simulink library "tqd"  (R2021b)
settings: Solver=VariableStepAuto  StartTime=0.0  StopTime=10.0  RelTol=1e-3
undefined symbols (not defined in the file or in its folder): ATQD_AccelLimitInRange_X_rpm, ATQD_AccelLimitInRange_Y_Nm, ATQD_AccelLimitOvrKi_X_Nm, ATQD_AccelLimitOvrKp_X_Nm, ATQD_BOSMapD_X_rpm, ATQD_BOSMapD_Y_pct, ATQD_BOSMapR_X_rpm, ATQD_BOSMapR_Y_pct, ATQD_HVBCurrSmooth_X_A, ATQD_LHMTqMapDLC_X_rpm, ATQD_LHMTqMapDLC_Y_pct, ATQD_LHMTqMapRLC_X_rpm, ATQD_LHMTqMapRLC_Y_pct, ATQD_NormalMapDLC_X_rpm, ATQD_NormalMapDLC_Y_pct, ATQD_NormalTqDecSR_X_rpm, ATQD_NormalTqDecSR_Y_Nm, ATQD_NormalTqIncSR_X_rpm, ATQD_NormalTqIncSR_Y_Nm, ATQD_OPDMapRLC_X_rpm, ATQD_OPDMapRLC_Y_pct, ATQD_RollRegTorReq_X_rpm, ATQD_RollRegTorReq_Y_enum, ATQD_VehSpdLimitInRange_X_rpm, ATQD_VehSpdLimitInRange_Y_Nm, ATQD_VehSpdLimitOvrKi_X_Nm, ATQD_VehSpdLimitOvrKp_X_Nm, EIGHT_INT, ENUM_BRAKEPEDAL_PRESSED, ENUM_BRAKEPEDAL_RELEASED, ENUM_COMBOKEY_DOWN, ENUM_COMBOKEY_M1, ENUM_COMBOKEY_M2, ENUM_COMBOKEY_NONE, ENUM_COMBOKEY_RKNEE, ENUM_COMBOKEY_STOPLV, ENUM_COMBOKEY_UP, ENUM_CP2VKNEEREQ_REQUEST, ENUM_CP2VNLVREQ_LEVEL1, ENUM_CP2VNLVREQ_LEVEL2, ENUM_CP2VNLVREQ_LOWER, ENUM_CP2VNLVREQ_STOPLV, ENUM_CP2VNLVREQ_UPPER, ENUM_CREEPIND_DISABLE, ENUM_CREEPIND_READY, ENUM_CREEPIND_RUNNING, ENUM_CREEPIND_WARNING, ENUM_DRIVELINERELEASE_RELEASE, ENUM_EBSTORQUERWQ_LIMIT, ENUM_EBSTORQUERWQ_TORQUE, ENUM_ECPVCUDRM_CONFORT, ENUM_ECPVCUDRM_ECO, ENUM_ECPVCUDRM_NORMAL, ENUM_ECPVCUDRM_NOTAVAILABLE, ENUM_EMTqModeDrvBrk_Accel, ENUM_EMTqModeDrvBrk_Brake, ENUM_EMTqModeDrvBrk_Coast, ENUM_ETC2ACTDRIVEDIR_BACKWARD, ENUM_ETC2ACTDRIVEDIR_FORWARD, ENUM_ETC2ACTDRIVEDIR_STILL ... (+341)
libraries: simulink x109, hcu_lib x67
(part 5 of 13)

== system tqd/TQD/OutpConvert/EVCU2 SCP ==
  BInpConvert_outputs : Inport
  Bus Selector1 : BusSelector  OutputSignals=VTQD_TMTqCapMot_Nm,VTQD_TMTqCapGen_Nm
  Constant1 : Constant  Value=EPS  OutDataTypeStr=single
  Constant143 : Constant  Value=KTQD_MCUMaxRefTorq_Nm
  Constant144 : Constant  Value=KTQD_MCUMaxRefTorq_Nm
  Constant5 : Constant  Value=EPS  OutDataTypeStr=single
  Data Type Conversion3 : DataTypeConversion  OutDataTypeStr=single
  Data Type Conversion96 : DataTypeConversion  OutDataTypeStr=single
  Divide4 : Product  Inputs=*/
  Divide5 : Product  Inputs=*/
  Fix4 : Rounding  Operator=round
  Fix5 : Rounding  Operator=round
  Gain1 : Gain  Gain=HUNDRED  ParamDataTypeStr=single
  Gain6 : Gain  Gain=HUNDRED  ParamDataTypeStr=single
  Max : MinMax  Function=max  Inputs=2
  Max1 : MinMax  Function=max  Inputs=2
  Saturation15 : Saturate  UpperLimit=100000  LowerLimit=1
      settings: AttributesFormatString=|
      | UpperLimit: %<UpperLimit>
      | LowerLimit: %<LowerLimit>
  Saturation16 : Saturate  UpperLimit=100000  LowerLimit=1
      settings: AttributesFormatString=|
      | UpperLimit: %<UpperLimit>
      | LowerLimit: %<LowerLimit>
  VTQD_EVCU2MaxTorqAvail_pct : Outport
  VTQD_EVCU2MinTorqAvail_pct : Outport  Port=2
  wires:
  Data Type Conversion96/1 -> [VTQD_EVCU2MaxTorqAvail_pct]  "VTQD_EVCU2MaxTorqAvail_pct"
  Data Type Conversion3/1 -> [VTQD_EVCU2MinTorqAvail_pct]  "VTQD_EVCU2MinTorqAvail_pct"
  Divide4/1 -> Gain6/1
  Fix5/1 -> Data Type Conversion3/1
  Constant144/1 -> Saturation16/1
  Fix4/1 -> Data Type Conversion96/1
  Gain6/1 -> Fix4/1
  Constant143/1 -> Saturation15/1
  BInpConvert_outputs/1 -> Bus Selector1/1
  Bus Selector1/1 -> [VTQD_TMTqCapMot_Nm]  "<VTQD_TMTqCapMot_Nm>"
  Bus Selector1/2 -> [VTQD_TMTqCapGen_Nm]  "<VTQD_TMTqCapGen_Nm>"
  Max/1 -> Divide4/2
  Saturation15/1 -> Max/1
  [VTQD_TMTqCapMot_Nm] -> Divide4/1
  Constant5/1 -> Max/2
  Saturation16/1 -> Max1/1
  Constant1/1 -> Max1/2
  Max1/1 -> Divide5/2
  [VTQD_TMTqCapGen_Nm] -> Divide5/1
  [VTQD_EVCU2MaxTorqAvail_pct] -> VTQD_EVCU2MaxTorqAvail_pct/1
  [VTQD_EVCU2MinTorqAvail_pct] -> VTQD_EVCU2MinTorqAvail_pct/1
  Divide5/1 -> Gain1/1
  Gain1/1 -> Fix5/1

== system tqd/TQD/OutpConvert/MCUCMD SCP ==
  BSCPIn_outputs : Inport
  BInpConvert_outputs : Inport  Port=2
  Bus Selector : BusSelector  OutputSignals=VTQD_BrkSWOn_flg
  Bus Selector1 : BusSelector  OutputSignals=VINP_TransReqGear_enum,VDMM_DTCDMSRCIncorrect_flg,VINP_CANMsgValidTC1_flg,VINP_ParkBrakeSW_flg
  Constant111 : Constant  Value=KTQD_VCUMCUDemSpd_rpm
  Constant14 : Constant  Value=ENUM_TARGETGEAR_REVERSE
  Constant156 : Constant  Value=ENUM_VCUMCUGEAR_D
  Constant157 : Constant  Value=ENUM_VCUMCUGEAR_R
  Constant159 : Constant  Value=ENUM_VCUMCUGEAR_N
  Constant190 : Constant  Value=ENUM_TARGETGEAR_NONE
  Constant191 : Constant  Value=ENUM_TARGETGEAR_NEUTRAL
  Constant192 : Constant  Value=ENUM_VCUMCUGEAR_INVAILD
  Constant5 : Constant  Value=ENUM_TARGETGEAR_DRIVE
  Constant58 : Constant  Value=KTQD_VCUMCUDemLoNegVal_rpm
  Constant66 : Constant  Value=ENUM_VCUMCUGEAR_N
  Constant89 : Constant  Value=ENUM_TARGETGEAR_ERROR
  Data Type Conversion : DataTypeConversion  OutDataTypeStr=boolean
  Data Type Conversion1 : DataTypeConversion  OutDataTypeStr=single
  Data Type Conversion2 : DataTypeConversion
  Data Type Conversion57 : DataTypeConversion  OutDataTypeStr=single
  Equal{22,24,27..29} (5 alike) : RelationalOperator  Operator===  OutDataTypeStr=boolean  RndMeth=Simplest
  NOT5 : Logic  Operator=NOT  AllPortsSameDT=off  OutDataTypeStr=boolean
  OR4 : Logic  Operator=OR  AllPortsSameDT=off  OutDataTypeStr=boolean
  OR5 : Logic  Operator=OR  AllPortsSameDT=off  OutDataTypeStr=boolean
  Switch{24,52..53,70..71} (5 alike) : Switch  Criteria=u2 ~= 0
      settings: AttributesFormatString=%<Criteria>
  Unit Delay2 : UnitDelay  InitialCondition=uint8(0)  SampleTime=-1  HasFrameUpgradeWarning=on
      settings: AttributesFormatString=%<InitialCondition>
  VTQD_VCUMCUDemLoNegVal_rpm : Outport
  VTQD_VCUMCUDemSpd_rpm : Outport  Port=2
  VTQD_VCUMCUGearSta_enum : Outport  Port=3
  VTQD_VCUMCUHandBrk_flg : Outport  Port=4
  VTQD_VCUMCUFootBrk_flg : Outport  Port=5
  wires:
  Switch52/1 -> Switch71/3
  Constant14/1 -> Equal24/2
  Equal29/1 -> OR4/2
  Equal22/1 -> Switch52/2
  Switch24/1 -> [VTQD_VCUMCUGearSta_enum], Unit Delay2/1  "VTQD_VCUMCUGearSta_enum"
  [VINP_TransReqGear_enum] -> Equal27/1
  Constant190/1 -> Equal28/2
  Equal27/1 -> OR5/2
  NOT5/1 -> OR5/1
  OR5/1 -> Switch71/2
  Equal28/1 -> OR4/1
  Constant5/1 -> Equal22/2
  Data Type Conversion57/1 -> [VTQD_VCUMCUDemSpd_rpm]  "VTQD_VCUMCUDemSpd_rpm"
  Constant191/1 -> Equal29/2
  [VINP_TransReqGear_enum] -> Equal29/1
  [VINP_CANMsgValidTC1_flg] -> NOT5/1
  [VINP_TransReqGear_enum] -> Equal22/1
  [VDMM_DTCDMSRCIncorrect_flg] -> Switch24/2
  Switch53/1 -> Switch52/3
  Constant111/1 -> Data Type Conversion57/1
  Switch71/1 -> Switch24/3
  Unit Delay2/1 -> Switch70/3
  Constant89/1 -> Equal27/2
  Constant156/1 -> Switch52/1
  Switch70/1 -> Switch53/3
  Constant159/1 -> Switch70/1
  OR4/1 -> Switch70/2
  Constant192/1 -> Switch71/1
  Equal24/1 -> Switch53/2
  [VINP_TransReqGear_enum] -> Equal28/1
  Constant58/1 -> Data Type Conversion1/1
  [VINP_TransReqGear_enum] -> Equal24/1
  Data Type Conversion1/1 -> [VTQD_VCUMCUDemLoNegVal_rpm]  "VTQD_VCUMCUDemLoNegVal_rpm"
  Constant157/1 -> Switch53/1
  Constant66/1 -> Switch24/1
  Bus Selector1/1 -> [VINP_TransReqGear_enum]  "<VINP_TransReqGear_enum>"
  BSCPIn_outputs/1 -> Bus Selector1/1
  Bus Selector1/2 -> [VDMM_DTCDMSRCIncorrect_flg]  "<VDMM_DTCDMSRCIncorrect_flg>"
  [VTQD_VCUMCUDemLoNegVal_rpm] -> VTQD_VCUMCUDemLoNegVal_rpm/1
  [VTQD_VCUMCUDemSpd_rpm] -> VTQD_VCUMCUDemSpd_rpm/1
  [VTQD_VCUMCUGearSta_enum] -> VTQD_VCUMCUGearSta_enum/1
  Bus Selector1/3 -> [VINP_CANMsgValidTC1_flg]  "<VINP_CANMsgValidTC1_flg>"
  Bus Selector1/4 -> [VINP_ParkBrakeSW_flg]  "<VINP_ParkBrakeSW_flg>"
  BInpConvert_outputs/1 -> Bus Selector/1
  Bus Selector/1 -> [VTQD_BrkSWOn_flg]  "<VTQD_BrkSWOn_flg>"
  [VINP_ParkBrakeSW_flg] -> Data Type Conversion/1
  Data Type Conversion/1 -> [VTQD_VCUMCUHandBrk_flg]  "VTQD_VCUMCUHandBrk_flg"
  [VTQD_BrkSWOn_flg] -> Data Type Conversion2/1
  Data Type Conversion2/1 -> [VTQD_VCUMCUFootBrk_flg]  "VTQD_VCUMCUFootBrk_flg"
  [VTQD_VCUMCUFootBrk_flg] -> VTQD_VCUMCUFootBrk_flg/1
  [VTQD_VCUMCUHandBrk_flg] -> VTQD_VCUMCUHandBrk_flg/1

== system tqd/TQD/OutpConvert/MSF SCP ==
  BInpConvert_outputs : Inport
  Bus Selector : BusSelector  OutputSignals=VTQD_ParkingProtectAction_flg
  Constant145 : Constant  Value=ENUM_VCUEBSHBSW_ACTIVE
  Constant181 : Constant  Value=ENUM_VCUEBSHBSW_PASSIVE
  Switch84 : Switch  Criteria=u2 ~= 0
      settings: AttributesFormatString=%<Criteria>
  VTQD_VCUEBSHBSw_enum : Outport
  wires:
  [VTQD_ParkingProtectAction_flg] -> Switch84/2
  Constant145/1 -> Switch84/1
  Switch84/1 -> [VTQD_VCUEBSHBSw_enum]  "VTQD_VCUEBSHBSw_enum"
  Constant181/1 -> Switch84/3
  BInpConvert_outputs/1 -> Bus Selector/1
  Bus Selector/1 -> [VTQD_ParkingProtectAction_flg]  "<VTQD_ParkingProtectAction_flg>"
  [VTQD_VCUEBSHBSw_enum] -> VTQD_VCUEBSHBSw_enum/1

== system tqd/TQD/OutpConvert/RC1 SCP ==
  Constant63 : Constant  Value=ZERO_INT  OutDataTypeStr=Inherit: Inherit via back propagation
  Constant64 : Constant  Value=FOUR_INT  OutDataTypeStr=single
  Constant65 : Constant  Value=KTQD_MCUMaxRefTorq_Nm
  Constant98 : Constant  Value=ZERO_FLOAT  OutDataTypeStr=single
  Data Type Conversion31 : DataTypeConversion  OutDataTypeStr=uint8
  Data Type Conversion32 : DataTypeConversion  OutDataTypeStr=uint8
  Data Type Conversion{33..43,58} (12 alike) : DataTypeConversion  OutDataTypeStr=single
  VTQD_RC1RetType_enum : Outport
  VTQD_RC1RetLocat_enum : Outport  Port=2
  VTQD_RC1RetCtrlMth_enum : Outport  Port=3
  VTQD_RC1RetSpdIdleP1_rpm : Outport  Port=4
  VTQD_RC1PctTrqIdleP1_pct : Outport  Port=5
  VTQD_RC1MaxRetSpdP2_rpm : Outport  Port=6
  VTQD_RC1RetSpdP2_pct : Outport  Port=7
  VTQD_RC1MaxRetSpdP3_rpm : Outport  Port=8
  VTQD_RC1PctTrqP3_pct : Outport  Port=9
  VTQD_RC1RetSpdP4_rpm : Outport  Port=10
  VTQD_RC1PctTrqP4_pct : Outport  Port=11
  VTQD_RC1RetSpdPekTrqP5_Nm : Outport  Port=12
  VTQD_RC1RefRetTrq_Nm : Outport  Port=13
  VTQD_RC1PctTrqPekTrqP5_pct : Outport  Port=14
  wires:
  Data Type Conversion33/1 -> VTQD_RC1RetCtrlMth_enum/1  "VTQD_RC1RetCtrlMth_enum"
  Data Type Conversion35/1 -> VTQD_RC1PctTrqIdleP1_pct/1  "VTQD_RC1PctTrqIdleP1_pct"
  Data Type Conversion32/1 -> VTQD_RC1RetLocat_enum/1  "VTQD_RC1RetLocat_enum"
  [DefaultValue16b] -> Data Type Conversion41/1
  [DefaultValue16b] -> Data Type Conversion34/1
  [DefaultValue16b] -> Data Type Conversion36/1
  Data Type Conversion39/1 -> VTQD_RC1RetSpdP4_rpm/1  "VTQD_RC1RetSpdP4_rpm"
  Data Type Conversion58/1 -> VTQD_RC1MaxRetSpdP3_rpm/1  "VTQD_RC1MaxRetSpdP3_rpm"
  [OfsetDefaultValue] -> Data Type Conversion37/1
  [OfsetDefaultValue] -> Data Type Conversion43/1
  Data Type Conversion42/1 -> VTQD_RC1RefRetTrq_Nm/1  "VTQD_RC1RefRetTrq_Nm"
  [OfsetDefaultValue] -> Data Type Conversion40/1
  [OfsetDefaultValue] -> Data Type Conversion38/1
  Data Type Conversion31/1 -> VTQD_RC1RetType_enum/1  "VTQD_RC1RetType_enum"
  Constant64/1 -> Data Type Conversion32/1
  Constant63/1 -> Data Type Conversion31/1
  [DefaultValue16b] -> Data Type Conversion39/1
  [DefaultValue8b] -> Data Type Conversion33/1
  [OfsetDefaultValue] -> Data Type Conversion35/1
  Data Type Conversion36/1 -> VTQD_RC1MaxRetSpdP2_rpm/1  "VTQD_RC1MaxRetSpdP2_rpm"
  [DefaultValue16b] -> Data Type Conversion58/1
  Data Type Conversion40/1 -> VTQD_RC1PctTrqP4_pct/1  "VTQD_RC1PctTrqP4_pct"
  Data Type Conversion38/1 -> VTQD_RC1PctTrqP3_pct/1  "VTQD_RC1PctTrqP3_pct"
  Data Type Conversion41/1 -> VTQD_RC1RetSpdPekTrqP5_Nm/1  "VTQD_RC1RetSpdPekTrqP5_Nm"
  Data Type Conversion37/1 -> VTQD_RC1RetSpdP2_pct/1  "VTQD_RC1RetSpdP2_pct"
  Data Type Conversion43/1 -> VTQD_RC1PctTrqPekTrqP5_pct/1  "VTQD_RC1PctTrqPekTrqP5_pct"
  Constant65/1 -> Data Type Conversion42/1
  Data Type Conversion34/1 -> VTQD_RC1RetSpdIdleP1_rpm/1  "VTQD_RC1RetSpdIdleP1_rpm"
  Constant98/1 -> [OfsetDefaultValue], [DefaultValue8b], [DefaultValue16b]

== system tqd/TQD/OutpConvert/TUpA Indication ==
  BInpConvert_outputs : Inport
  Bus Selector : BusSelector  OutputSignals=VTQD_ComboKeyEn_flg,VTQD_ActTUpAIND_enum
  Constant19 : Constant  Value=ENUM_TUPAIND_RUNNING
  Switch1 : Switch  Criteria=u2 ~= 0
      settings: AttributesFormatString=%<Criteria>
  VTQD_TUpAIND_enum : Outport
  wires:
  Constant19/1 -> Switch1/1
  [VTQD_ActTUpAIND_enum] -> Switch1/3
  Switch1/1 -> [VTQD_TUpAIND_enum]  "VTQD_TUpAIND_enum"
  [VTQD_ComboKeyEn_flg] -> Switch1/2
  Bus Selector/1 -> [VTQD_ComboKeyEn_flg]  "<VTQD_ComboKeyEn_flg>"
  BInpConvert_outputs/1 -> Bus Selector/1
  Bus Selector/2 -> [VTQD_ActTUpAIND_enum]  "<VTQD_ActTUpAIND_enum>"
  [VTQD_TUpAIND_enum] -> VTQD_TUpAIND_enum/1

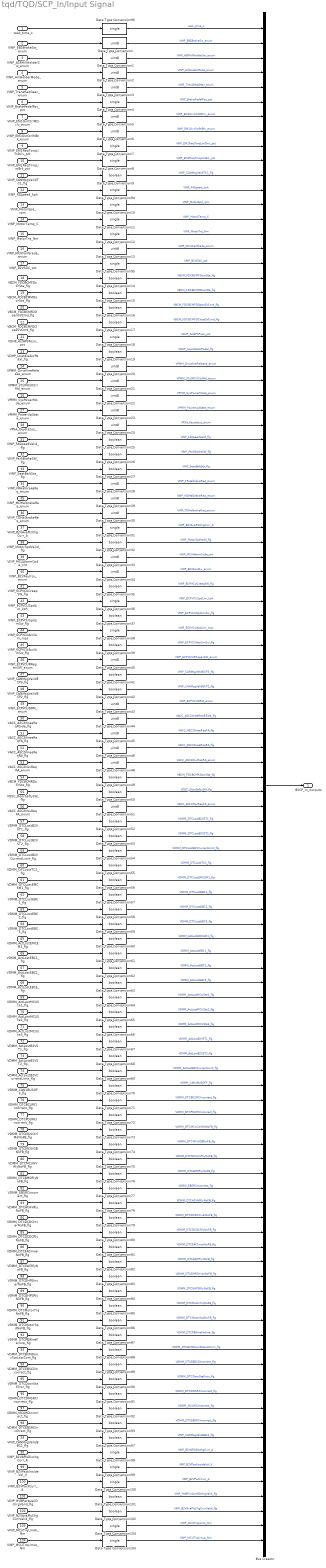
== system tqd/TQD/SCP_In/Input Signal ==
  task_time_s : Inport
  VINP_EBSBrakeSw_enum : Inport  Port=2
  VINP_ASRHillHolderSw_enum : Inport  Port=3
  VINP_HillHolderMode_enum : Inport  Port=4
  VINP_TransReqGear_enum : Inport  Port=5
  VINP_BrakePedalPos_pct : Inport  Port=6
  VINP_EM1OvrCtrlMDriv_enum : Inport  Port=7
  VINP_EM1OvrCtrlMBrk_enum : Inport  Port=8
  VINP_EM1ReqTorqLimDriv_pct : Inport  Port=9
  VINP_EM1ReqTorqLimBrk_pct : Inport  Port=10
  VINP_CANMsgValidTC1_flg : Inport  Port=11
  VINP_FASpeed_kph : Inport  Port=12
  VINP_MotorSpd_rpm : Inport  Port=13
  VINP_MotorTemp_C : Inport  Port=14
  VINP_MotorTrq_Nm : Inport  Port=15
  VINP_MCUFailGrade_enum : Inport  Port=16
  VINP_B2VSOC_pct : Inport  Port=17
  VBCM_FDCBCMFDoorSta_flg : Inport  Port=18
  VBCM_FDCBCMMDoorSta_flg : Inport  Port=19
  VBCM_FDCBCMFDOpenSVCmd_flg : Inport  Port=20
  VBCM_FDCBCMFDCloseSVCmd_flg : Inport  Port=21
  VDHP_ActAPSPosn_pct : Inport  Port=22
  VDHP_LowIdleAccPedal_flg : Inport  Port=23
  VPMM_DrivelineRelease_enum : Inport  Port=24
  VPMM_VCUMCUCtrlMd_enum : Inport  Port=25
  VPMM_SysPowerMode_enum : Inport  Port=26
  VPMM_PowerUpState_enum : Inport  Port=27
  VPSA_Keystatus_enum : Inport  Port=28
  VINP_CANMsgValidEBC2_flg : Inport  Port=29
  VINP_B2VAPlsDischgCurr_A : Inport  Port=30
  VINP_FASpeedValid_flg : Inport  Port=31
  VINP_ParkBrakeSW_flg : Inport  Port=32
  VINP_SeatBeltSta_flg : Inport  Port=33
  VINP_FRHalbrakeReq_enum : Inport  Port=34
  VINP_MDHalbrakeReq_enum : Inport  Port=35
  VINP_TDHalbrakeReq_enum : Inport  Port=36
  VINP_B2VAvaPlsChgCurr_A : Inport  Port=37
  VINP_MotorSpdValid_flg : Inport  Port=38
  VINP_MCUAlarmCode_cnt : Inport  Port=39
  VINP_B2VFaultLv_enum : Inport  Port=40
  VINP_ECPVCUCreepSW_flg : Inport  Port=41
  VINP_ECPVCUSpdLim_kph : Inport  Port=42
  VINP_ECPVCUSpdLimSw_flg : Inport  Port=43
  VINP_ECPVCUAcclLim_mps : Inport  Port=44
  VINP_ECPVCUAcclLimSw_flg : Inport  Port=45
  VINP_ECPVCURRegenSW_enum : Inport  Port=46
  VINP_CANMsgValidECP3_flg : Inport  Port=47
  VINP_CANMsgValidECP2_flg : Inport  Port=48
  VINP_ECPVCUDRM_enum : Inport  Port=49
  VACC_ASC2KneeReqRSide_flg : Inport  Port=50
  VACC_ASC2KneeReqFA_flg : Inport  Port=51
  VACC_ASC2KneeReqRA_flg : Inport  Port=52
  VACC_ASC2NLvReqRA_enum : Inport  Port=53
  VBCM_FDCBCMRDoorSta_flg : Inport  Port=54
  VDSC_DoorSaftySW_flg : Inport  Port=55
  VACC_ASC2NLvReqFA_enum : Inport  Port=56
  VDMM_DTCLostB2VST1_flg : Inport  Port=57
  VDMM_DTCLostB2VST2_flg : Inport  Port=58
  VDMM_DTCLostB2VCurrentLimit_flg : Inport  Port=59
  VDMM_DTCLostTC1_flg : Inport  Port=60
  VDMM_DTCLostEMCEM1_flg : Inport  Port=61
  VDMM_DTCLostEBC1_flg : Inport  Port=62
  VDMM_DTCLostEBC2_flg : Inport  Port=63
  VDMM_DTCLostEBC5_flg : Inport  Port=64
  VDMM_ActLostEMCEM1_flg : Inport  Port=65
  VDMM_ActLostEBC1_flg : Inport  Port=66
  VDMM_ActLostEBC2_flg : Inport  Port=67
  VDMM_ActLostEBC5_flg : Inport  Port=68
  VDMM_ActLostMCUSta1_flg : Inport  Port=69
  VDMM_ActLostMCUSta2_flg : Inport  Port=70
  VDMM_ActLostMCUSta3_flg : Inport  Port=71
  VDMM_ActLostB2VST1_flg : Inport  Port=72
  VDMM_ActLostB2VST2_flg : Inport  Port=73
  VDMM_ActLostB2VCurrentLimit_flg : Inport  Port=74
  VDMM_CAN1BUSOFF_flg : Inport  Port=75
  VDMM_DTCBCURCIncorrect_flg : Inport  Port=76
  VDMM_DTCPDURCIncorrect_flg : Inport  Port=77
  VDMM_DTCMCUCtrlMdNoFB_flg : Inport  Port=78
  VDMM_DTCMCUIGBNoFB_flg : Inport  Port=79
  VDMM_DTCMCUHVRlyNoFB_flg : Inport  Port=80
  VDMM_DTCBMSRlyNoFB_flg : Inport  Port=81
  VDMM_EBSRCIncorrect_flg : Inport  Port=82
  VDMM_DTCACHVRlyNoFB_flg : Inport  Port=83
  VDMM_DTCDCDCInverNoFB_flg : Inport  Port=84
  VDMM_DTCDCDCRlyNoFB_flg : Inport  Port=85
  VDMM_DTCEACInverNoFB_flg : Inport  Port=86
  VDMM_DTCEACRlyNoFB_flg : Inport  Port=87
  VDMM_DTCEHPSInverNoFB_flg : Inport  Port=88
  VDMM_DTCEHPSRlyNoFB_flg : Inport  Port=89
  VDMM_DTCMotorTrqNoFB_flg : Inport  Port=90
  VDMM_DTCMotorSpdNoFB_flg : Inport  Port=91
  VDMM_DTCPBWireFailure_flg : Inport  Port=92
  VDMM_DTCBCMDoorStaLostCom_flg : Inport  Port=93
  VDMM_DTCEBSCSIncorrect_flg : Inport  Port=94
  VDMM_DTCDoorStaError_flg : Inport  Port=95
  VDMM_DTCDMSRCIncorrect_flg : Inport  Port=96
  VDMM_MCURCIncorrect_flg : Inport  Port=97
  VDMM_DTCEBSRCIncorrect_flg : Inport  Port=98
  VINP_B2VPackInsideVol_V : Inport  Port=99
  VINP_B2VPackCurr_A : Inport  Port=100
  VINP_HVBPwrAvailDchrgValid_flg : Inport  Port=101
  VINP_B2VAvaPlsChgCurrValid_flg : Inport  Port=102
  VINP_MCUTrqLimHi_Nm : Inport  Port=103
  VINP_MCUTrqLimLo_Nm : Inport  Port=104
  Bus Creator : BusCreator  Inputs=104
  Data Type Conversion{,1..3,5..6,13,20..24,28..30,33..34,40,43..46,48,51} (24 alike) : DataTypeConversion  OutDataTypeStr=uint8
  Data Type Conversion{4,7..8,10..12,18,31,36,38,94..96,98..100,103..104} (18 alike) : DataTypeConversion  OutDataTypeStr=single
  Data Type Conversion{9,14..17,19,25..27,32,35,37,39,41..42,49..50,52..93,97,101..102} (62 alike) : DataTypeConversion  OutDataTypeStr=boolean
  BSCP_In_outputs : Outport
  wires:
  VINP_ECPVCUAcclLim_mps/1 -> Data Type Conversion38/1
  VDMM_DTCBCMDoorStaLostCom_flg/1 -> Data Type Conversion88/1
  Data Type Conversion30/1 -> Bus Creator/34  "VINP_TDHalbrakeReq_enum"
  VINP_SeatBeltSta_flg/1 -> Data Type Conversion27/1
  Data Type Conversion29/1 -> Bus Creator/33  "VINP_MDHalbrakeReq_enum"
  VINP_MDHalbrakeReq_enum/1 -> Data Type Conversion29/1
  Data Type Conversion94/1 -> Bus Creator/12  "VINP_FASpeed_kph"
  VDMM_DTCDCDCRlyNoFB_flg/1 -> Data Type Conversion80/1
  Data Type Conversion20/1 -> Bus Creator/24  "VPMM_DrivelineRelease_enum"
  VDMM_DTCDoorStaError_flg/1 -> Data Type Conversion90/1
  Data Type Conversion14/1 -> Bus Creator/18  "VBCM_FDCBCMFDoorSta_flg"
  Data Type Conversion3/1 -> Bus Creator/5  "VINP_TransReqGear_enum"
  VINP_EBSBrakeSw_enum/1 -> Data Type Conversion/1
  Data Type Conversion6/1 -> Bus Creator/8  "VINP_EM1OvrCtrlMBrk_enum"
  VINP_EM1OvrCtrlMBrk_enum/1 -> Data Type Conversion6/1
  VPMM_SysPowerMode_enum/1 -> Data Type Conversion22/1
  Data Type Conversion38/1 -> Bus Creator/42  "VINP_ECPVCUAcclLim_mps"
  VDMM_DTCDCDCInverNoFB_flg/1 -> Data Type Conversion79/1
  Data Type Conversion43/1 -> Bus Creator/47  "VINP_ECPVCUDRM_enum"
  Data Type Conversion18/1 -> Bus Creator/22  "VDHP_ActAPSPosn_pct"
  Data Type Conversion46/1 -> Bus Creator/50  "VACC_ASC2KneeReqRA_flg"
  Data Type Conversion16/1 -> Bus Creator/20  "VBCM_FDCBCMFDOpenSVCmd_flg"
  VPSA_Keystatus_enum/1 -> Data Type Conversion24/1
  VDMM_DTCMotorSpdNoFB_flg/1 -> Data Type Conversion86/1
  Data Type Conversion45/1 -> Bus Creator/49  "VACC_ASC2KneeReqFA_flg"
  VDMM_DTCPDURCIncorrect_flg/1 -> Data Type Conversion72/1
  Data Type Conversion5/1 -> Bus Creator/7  "VINP_EM1OvrCtrlMDriv_enum"
  Data Type Conversion22/1 -> Bus Creator/26  "VPMM_SysPowerMode_enum"
  VDMM_ActLostEBC1_flg/1 -> Data Type Conversion61/1
  Data Type Conversion35/1 -> Bus Creator/39  "VINP_ECPVCUCreepSW_flg"
  VINP_MCUAlarmCode_cnt/1 -> Data Type Conversion33/1
  Data Type Conversion34/1 -> Bus Creator/38  "VINP_B2VFaultLv_enum"
  Data Type Conversion19/1 -> Bus Creator/23  "VDHP_LowIdleAccPedal_flg"
  Data Type Conversion1/1 -> Bus Creator/3  "VINP_ASRHillHolderSw_enum"
  Data Type Conversion15/1 -> Bus Creator/19  "VBCM_FDCBCMMDoorSta_flg"
  VINP_CANMsgValidECP2_flg/1 -> Data Type Conversion42/1
  VDSC_DoorSaftySW_flg/1 -> Data Type Conversion50/1
  Data Type Conversion33/1 -> Bus Creator/37  "VINP_MCUAlarmCode_cnt"
  Data Type Conversion96/1 -> Bus Creator/1  "task_time_s"
  VDMM_DTCEHPSInverNoFB_flg/1 -> Data Type Conversion83/1
  VINP_FASpeed_kph/1 -> Data Type Conversion94/1
  VACC_ASC2NLvReqRA_enum/1 -> Data Type Conversion48/1
  VINP_ECPVCUSpdLim_kph/1 -> Data Type Conversion36/1
  Data Type Conversion12/1 -> Bus Creator/15  "VINP_MotorTrq_Nm"
  VINP_HillHolderMode_enum/1 -> Data Type Conversion2/1
  VDHP_LowIdleAccPedal_flg/1 -> Data Type Conversion19/1
  Data Type Conversion36/1 -> Bus Creator/40  "VINP_ECPVCUSpdLim_kph"
  Data Type Conversion37/1 -> Bus Creator/41  "VINP_ECPVCUSpdLimSw_flg"
  Data Type Conversion17/1 -> Bus Creator/21  "VBCM_FDCBCMFDCloseSVCmd_flg"
  Data Type Conversion4/1 -> Bus Creator/6  "VINP_BrakePedalPos_pct"
  VDMM_MCURCIncorrect_flg/1 -> Data Type Conversion92/1
  Data Type Conversion9/1 -> Bus Creator/11  "VINP_CANMsgValidTC1_flg"
  Data Type Conversion95/1 -> Bus Creator/17  "VINP_B2VSOC_pct"
  Data Type Conversion21/1 -> Bus Creator/25  "VPMM_VCUMCUCtrlMd_enum"
  Data Type Conversion42/1 -> Bus Creator/46  "VINP_CANMsgValidECP2_flg"
  Data Type Conversion39/1 -> Bus Creator/43  "VINP_ECPVCUAcclLimSw_flg"
  Data Type Conversion28/1 -> Bus Creator/32  "VINP_FRHalbrakeReq_enum"
  VBCM_FDCBCMFDCloseSVCmd_flg/1 -> Data Type Conversion17/1
  Data Type Conversion8/1 -> Bus Creator/10  "VINP_EM1ReqTorqLimBrk_pct"
  Data Type Conversion40/1 -> Bus Creator/44  "VINP_ECPVCURRegenSW_enum"
  VDMM_DTCEACRlyNoFB_flg/1 -> Data Type Conversion82/1
  Data Type Conversion/1 -> Bus Creator/2  "VINP_EBSBrakeSw_enum"
  VBCM_FDCBCMFDoorSta_flg/1 -> Data Type Conversion14/1
  Data Type Conversion24/1 -> Bus Creator/28  "VPSA_Keystatus_enum"
  Data Type Conversion23/1 -> Bus Creator/27  "VPMM_PowerUpState_enum"
  Data Type Conversion7/1 -> Bus Creator/9  "VINP_EM1ReqTorqLimDriv_pct"
  Data Type Conversion32/1 -> Bus Creator/36  "VINP_MotorSpdValid_flg"
  Data Type Conversion10/1 -> Bus Creator/13  "VINP_MotorSpd_rpm"
  VDMM_CAN1BUSOFF_flg/1 -> Data Type Conversion70/1
  Data Type Conversion44/1 -> Bus Creator/48  "VACC_ASC2KneeReqRSide_flg"
  VINP_ASRHillHolderSw_enum/1 -> Data Type Conversion1/1
  VINP_ECPVCUDRM_enum/1 -> Data Type Conversion43/1
  VBCM_FDCBCMMDoorSta_flg/1 -> Data Type Conversion15/1
  Data Type Conversion31/1 -> Bus Creator/35  "VINP_B2VAvaPlsChgCurr_A"
  Data Type Conversion26/1 -> Bus Creator/30  "VINP_ParkBrakeSW_flg"
  Data Type Conversion25/1 -> Bus Creator/29  "VINP_FASpeedValid_flg"
  Data Type Conversion41/1 -> Bus Creator/45  "VINP_CANMsgValidECP3_flg"
  VINP_ECPVCUSpdLimSw_flg/1 -> Data Type Conversion37/1
  Data Type Conversion27/1 -> Bus Creator/31  "VINP_SeatBeltSta_flg"
  Bus Creator/1 -> BSCP_In_outputs/1
  Data Type Conversion11/1 -> Bus Creator/14  "VINP_MotorTemp_C"
  Data Type Conversion2/1 -> Bus Creator/4  "VINP_HillHolderMode_enum"
  Data Type Conversion13/1 -> Bus Creator/16  "VINP_MCUFailGrade_enum"
  VDMM_DTCMCUCtrlMdNoFB_flg/1 -> Data Type Conversion73/1
  VINP_ParkBrakeSW_flg/1 -> Data Type Conversion26/1
  VDMM_DTCMCUHVRlyNoFB_flg/1 -> Data Type Conversion75/1
  VDMM_DTCLostB2VST2_flg/1 -> Data Type Conversion53/1
  VDMM_ActLostMCUSta3_flg/1 -> Data Type Conversion66/1
  VDMM_ActLostEMCEM1_flg/1 -> Data Type Conversion60/1
  VBCM_FDCBCMRDoorSta_flg/1 -> Data Type Conversion49/1
  VINP_TransReqGear_enum/1 -> Data Type Conversion3/1
  VACC_ASC2KneeReqRA_flg/1 -> Data Type Conversion46/1
  VDMM_DTCEBSCSIncorrect_flg/1 -> Data Type Conversion89/1
  VINP_EM1ReqTorqLimBrk_pct/1 -> Data Type Conversion8/1
  VINP_EM1ReqTorqLimDriv_pct/1 -> Data Type Conversion7/1
  VPMM_DrivelineRelease_enum/1 -> Data Type Conversion20/1
  VDMM_DTCDMSRCIncorrect_flg/1 -> Data Type Conversion91/1
  VINP_FRHalbrakeReq_enum/1 -> Data Type Conversion28/1
  VDMM_DTCMCUIGBNoFB_flg/1 -> Data Type Conversion74/1
  VINP_EM1OvrCtrlMDriv_enum/1 -> Data Type Conversion5/1
  VINP_MotorSpdValid_flg/1 -> Data Type Conversion32/1
  VINP_ECPVCUCreepSW_flg/1 -> Data Type Conversion35/1
  VDMM_DTCLostEBC1_flg/1 -> Data Type Conversion57/1
  VDMM_ActLostB2VST2_flg/1 -> Data Type Conversion68/1
  VINP_FASpeedValid_flg/1 -> Data Type Conversion25/1
  VDMM_DTCEHPSRlyNoFB_flg/1 -> Data Type Conversion84/1
  VDMM_DTCMotorTrqNoFB_flg/1 -> Data Type Conversion85/1
  VINP_CANMsgValidTC1_flg/1 -> Data Type Conversion9/1
  VDMM_DTCEBSRCIncorrect_flg/1 -> Data Type Conversion93/1
  VDMM_DTCPBWireFailure_flg/1 -> Data Type Conversion87/1
  VPMM_PowerUpState_enum/1 -> Data Type Conversion23/1
  VPMM_VCUMCUCtrlMd_enum/1 -> Data Type Conversion21/1
  VINP_B2VSOC_pct/1 -> Data Type Conversion95/1
  VDMM_EBSRCIncorrect_flg/1 -> Data Type Conversion77/1
  VDMM_ActLostB2VCurrentLimit_flg/1 -> Data Type Conversion69/1
  VACC_ASC2KneeReqRSide_flg/1 -> Data Type Conversion44/1
  VACC_ASC2KneeReqFA_flg/1 -> Data Type Conversion45/1
  VDMM_DTCLostB2VST1_flg/1 -> Data Type Conversion52/1
  VDMM_DTCACHVRlyNoFB_flg/1 -> Data Type Conversion78/1
  VDMM_DTCLostTC1_flg/1 -> Data Type Conversion55/1
  VINP_ECPVCUAcclLimSw_flg/1 -> Data Type Conversion39/1
  VINP_CANMsgValidECP3_flg/1 -> Data Type Conversion41/1
  VDMM_DTCLostEBC2_flg/1 -> Data Type Conversion58/1
  VACC_ASC2NLvReqFA_enum/1 -> Data Type Conversion51/1
  VINP_B2VAvaPlsChgCurr_A/1 -> Data Type Conversion31/1
  VDMM_ActLostMCUSta2_flg/1 -> Data Type Conversion65/1
  VDMM_ActLostEBC2_flg/1 -> Data Type Conversion62/1
  VDMM_ActLostMCUSta1_flg/1 -> Data Type Conversion64/1
  VDMM_ActLostB2VST1_flg/1 -> Data Type Conversion67/1
  VINP_MCUFailGrade_enum/1 -> Data Type Conversion13/1
  VDMM_DTCLostEBC5_flg/1 -> Data Type Conversion59/1
  VBCM_FDCBCMFDOpenSVCmd_flg/1 -> Data Type Conversion16/1
  VDHP_ActAPSPosn_pct/1 -> Data Type Conversion18/1
  VDMM_ActLostEBC5_flg/1 -> Data Type Conversion63/1
  VINP_BrakePedalPos_pct/1 -> Data Type Conversion4/1
  VDMM_DTCBCURCIncorrect_flg/1 -> Data Type Conversion71/1
  VINP_B2VFaultLv_enum/1 -> Data Type Conversion34/1
  VDMM_DTCEACInverNoFB_flg/1 -> Data Type Conversion81/1
  VINP_TDHalbrakeReq_enum/1 -> Data Type Conversion30/1
  VDMM_DTCLostEMCEM1_flg/1 -> Data Type Conversion56/1
  VINP_MotorSpd_rpm/1 -> Data Type Conversion10/1
  VINP_ECPVCURRegenSW_enum/1 -> Data Type Conversion40/1
  VINP_MotorTemp_C/1 -> Data Type Conversion11/1
  VDMM_DTCLostB2VCurrentLimit_flg/1 -> Data Type Conversion54/1
  VDMM_DTCBMSRlyNoFB_flg/1 -> Data Type Conversion76/1
  VINP_MotorTrq_Nm/1 -> Data Type Conversion12/1
  task_time_s/1 -> Data Type Conversion96/1
  VINP_CANMsgValidEBC2_flg/1 -> Data Type Conversion97/1
  VINP_B2VAPlsDischgCurr_A/1 -> Data Type Conversion98/1
  VINP_B2VAvaPlsChgCurrValid_flg/1 -> Data Type Conversion102/1
  VINP_HVBPwrAvailDchrgValid_flg/1 -> Data Type Conversion101/1
  VINP_B2VPackInsideVol_V/1 -> Data Type Conversion99/1
  VINP_B2VPackCurr_A/1 -> Data Type Conversion100/1
  VINP_MCUTrqLimLo_Nm/1 -> Data Type Conversion103/1
  VINP_MCUTrqLimHi_Nm/1 -> Data Type Conversion104/1
  Data Type Conversion48/1 -> Bus Creator/51  "VACC_ASC2NLvReqRA_enum"
  Data Type Conversion49/1 -> Bus Creator/52  "VBCM_FDCBCMRDoorSta_flg"
  Data Type Conversion50/1 -> Bus Creator/53  "VDSC_DoorSaftySW_flg"
  Data Type Conversion51/1 -> Bus Creator/54  "VACC_ASC2NLvReqFA_enum"
  Data Type Conversion52/1 -> Bus Creator/55  "VDMM_DTCLostB2VST1_flg"
  Data Type Conversion53/1 -> Bus Creator/56  "VDMM_DTCLostB2VST2_flg"
  Data Type Conversion54/1 -> Bus Creator/57  "VDMM_DTCLostB2VCurrentLimit_flg"
  Data Type Conversion55/1 -> Bus Creator/58  "VDMM_DTCLostTC1_flg"
  Data Type Conversion56/1 -> Bus Creator/59  "VDMM_DTCLostEMCEM1_flg"
  Data Type Conversion57/1 -> Bus Creator/60  "VDMM_DTCLostEBC1_flg"
  Data Type Conversion58/1 -> Bus Creator/61  "VDMM_DTCLostEBC2_flg"
  Data Type Conversion59/1 -> Bus Creator/62  "VDMM_DTCLostEBC5_flg"
  Data Type Conversion60/1 -> Bus Creator/63  "VDMM_ActLostEMCEM1_flg"
  Data Type Conversion61/1 -> Bus Creator/64  "VDMM_ActLostEBC1_flg"
  Data Type Conversion62/1 -> Bus Creator/65  "VDMM_ActLostEBC2_flg"
  Data Type Conversion63/1 -> Bus Creator/66  "VDMM_ActLostEBC5_flg"
  Data Type Conversion64/1 -> Bus Creator/67  "VDMM_ActLostMCUSta1_flg"
  Data Type Conversion65/1 -> Bus Creator/68  "VDMM_ActLostMCUSta2_flg"
  Data Type Conversion66/1 -> Bus Creator/69  "VDMM_ActLostMCUSta3_flg"
  Data Type Conversion67/1 -> Bus Creator/70  "VDMM_ActLostB2VST1_flg"
  Data Type Conversion68/1 -> Bus Creator/71  "VDMM_ActLostB2VST2_flg"
  Data Type Conversion69/1 -> Bus Creator/72  "VDMM_ActLostB2VCurrentLimit_flg"
  Data Type Conversion70/1 -> Bus Creator/73  "VDMM_CAN1BUSOFF_flg"
  Data Type Conversion71/1 -> Bus Creator/74  "VDMM_DTCBCURCIncorrect_flg"
  Data Type Conversion72/1 -> Bus Creator/75  "VDMM_DTCPDURCIncorrect_flg"
  Data Type Conversion73/1 -> Bus Creator/76  "VDMM_DTCMCUCtrlMdNoFB_flg"
  Data Type Conversion74/1 -> Bus Creator/77  "VDMM_DTCMCUIGBNoFB_flg"
  Data Type Conversion75/1 -> Bus Creator/78  "VDMM_DTCMCUHVRlyNoFB_flg"
  Data Type Conversion76/1 -> Bus Creator/79  "VDMM_DTCBMSRlyNoFB_flg"
  Data Type Conversion77/1 -> Bus Creator/80  "VDMM_EBSRCIncorrect_flg"
  Data Type Conversion78/1 -> Bus Creator/81  "VDMM_DTCACHVRlyNoFB_flg"
  Data Type Conversion79/1 -> Bus Creator/82  "VDMM_DTCDCDCInverNoFB_flg"
  Data Type Conversion80/1 -> Bus Creator/83  "VDMM_DTCDCDCRlyNoFB_flg"
  Data Type Conversion81/1 -> Bus Creator/84  "VDMM_DTCEACInverNoFB_flg"
  Data Type Conversion82/1 -> Bus Creator/85  "VDMM_DTCEACRlyNoFB_flg"
  Data Type Conversion83/1 -> Bus Creator/86  "VDMM_DTCEHPSInverNoFB_flg"
  Data Type Conversion84/1 -> Bus Creator/87  "VDMM_DTCEHPSRlyNoFB_flg"
  Data Type Conversion85/1 -> Bus Creator/88  "VDMM_DTCMotorTrqNoFB_flg"
  Data Type Conversion86/1 -> Bus Creator/89  "VDMM_DTCMotorSpdNoFB_flg"
  Data Type Conversion87/1 -> Bus Creator/90  "VDMM_DTCPBWireFailure_flg"
  Data Type Conversion88/1 -> Bus Creator/91  "VDMM_DTCBCMDoorStaLostCom_flg"
  Data Type Conversion89/1 -> Bus Creator/92  "VDMM_DTCEBSCSIncorrect_flg"
  Data Type Conversion90/1 -> Bus Creator/93  "VDMM_DTCDoorStaError_flg"
  Data Type Conversion91/1 -> Bus Creator/94  "VDMM_DTCDMSRCIncorrect_flg"
  Data Type Conversion92/1 -> Bus Creator/95  "VDMM_MCURCIncorrect_flg"
  Data Type Conversion93/1 -> Bus Creator/96  "VDMM_DTCEBSRCIncorrect_flg"
  Data Type Conversion97/1 -> Bus Creator/97  "VINP_CANMsgValidEBC2_flg"
  Data Type Conversion98/1 -> Bus Creator/98  "VINP_B2VAPlsDischgCurr_A"
  Data Type Conversion99/1 -> Bus Creator/99  "VINP_B2VPackInsideVol_V"
  Data Type Conversion100/1 -> Bus Creator/100  "VINP_B2VPackCurr_A"
  Data Type Conversion101/1 -> Bus Creator/101  "VINP_HVBPwrAvailDchrgValid_flg"
  Data Type Conversion102/1 -> Bus Creator/102  "VINP_B2VAvaPlsChgCurrValid_flg"
  Data Type Conversion104/1 -> Bus Creator/103  "VINP_MCUTrqLimHi_Nm"
  Data Type Conversion103/1 -> Bus Creator/104  "VINP_MCUTrqLimLo_Nm"

== system tqd/TQD/SCP_In/Invalid Condition ==
  VDMM_MCURCIncorrect_flg : Inport
  VINP_FASpeedValid_flg : Inport  Port=2
  VDMM_DTCDMSRCIncorrect_flg : Inport  Port=3
  VDMM_DTCEBSRCIncorrect_flg : Inport  Port=4
  VINP_MotorSpdValid_flg : Inport  Port=5
  Bus Creator : BusCreator  Inputs=10
  Data Type Conversion{,1..9} (10 alike) : DataTypeConversion  OutDataTypeStr=boolean
  NOT : Logic  Operator=NOT  AllPortsSameDT=off  OutDataTypeStr=boolean
  NOT1 : Logic  Operator=NOT  AllPortsSameDT=off  OutDataTypeStr=boolean
  OR : Logic  Operator=OR  AllPortsSameDT=off  OutDataTypeStr=boolean
  BDCQ_SCPInInValid_outputs : Outport
  wires:
  Data Type Conversion1/1 -> Bus Creator/2  "VTQD_FASpeedInV_flg"
  [VINP_FASpeedValid_flg] -> NOT/1
  Data Type Conversion/1 -> Bus Creator/1  "VTQD_MotorSpdInV_flg"
  Bus Creator/1 -> BDCQ_SCPInInValid_outputs/1
  VDMM_MCURCIncorrect_flg/1 -> [VDMM_MCURCIncorrect_flg]
  VINP_FASpeedValid_flg/1 -> [VINP_FASpeedValid_flg]
  NOT/1 -> Data Type Conversion1/1
  VDMM_DTCDMSRCIncorrect_flg/1 -> [VDMM_DTCDMSRCIncorrect_flg]
  [VDMM_DTCDMSRCIncorrect_flg] -> Data Type Conversion2/1
  Data Type Conversion2/1 -> Bus Creator/3  "VTQD_TransReqGearInV_flg"
  [VDMM_MCURCIncorrect_flg] -> Data Type Conversion3/1
  Data Type Conversion3/1 -> Bus Creator/4  "VTQD_MotorTempInV_flg"
  [VDMM_MCURCIncorrect_flg] -> Data Type Conversion4/1
  Data Type Conversion4/1 -> Bus Creator/5  "VTQD_MotorTrqInV_flg"
  VDMM_DTCEBSRCIncorrect_flg/1 -> [VDMM_DTCEBSRCIncorrect_flg]
  [VDMM_DTCEBSRCIncorrect_flg] -> Data Type Conversion5/1
  Data Type Conversion5/1 -> Bus Creator/6  "VTQD_EM1OvrCtrlMDrivInV_flg"
  [VDMM_DTCEBSRCIncorrect_flg] -> Data Type Conversion6/1
  Data Type Conversion6/1 -> Bus Creator/7  "VTQD_EM1OvrCtrlMBrkInV_flg"
  [VDMM_DTCEBSRCIncorrect_flg] -> Data Type Conversion7/1
  Data Type Conversion7/1 -> Bus Creator/8  "VTQD_EM1ReqTorqLimDrivInV_flg"
  [VDMM_DTCEBSRCIncorrect_flg] -> Data Type Conversion8/1
  Data Type Conversion8/1 -> Bus Creator/9  "VTQD_EM1ReqTorqLimBrkInV_flg"
  VINP_MotorSpdValid_flg/1 -> [VINP_MotorSpdValid_flg]
  OR/1 -> Data Type Conversion/1
  [VDMM_MCURCIncorrect_flg] -> OR/1
  NOT1/1 -> OR/2
  [VINP_MotorSpdValid_flg] -> NOT1/1
  [VDMM_DTCEBSRCIncorrect_flg] -> Data Type Conversion9/1
  Data Type Conversion9/1 -> Bus Creator/10  "VTQD_MCUFailGradeInV_flg"

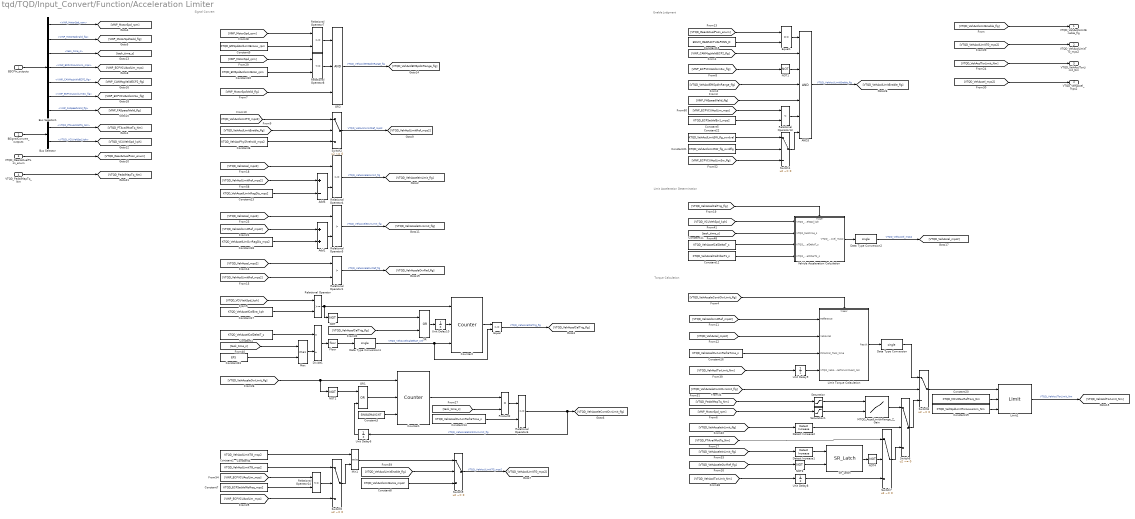
== system tqd/TQD/Input_Convert/Function/Acceleration Limiter ==
  note: Torque Calculation
  note: Limit Acceleration Determination
  note: Enable Judgment
  note: Signal Convert
  BSCPIn_outputs : Inport
  BSignalConvert_outputs : Inport  Port=2
  VTQD_GearActualPosn_enum : Inport  Port=3
  VTQD_PedalMapTq_Nm : Inport  Port=4
  AND3 : Logic  Inputs=7  AllPortsSameDT=off  OutDataTypeStr=boolean
  Add1 : Sum
  Add6 : Sum  Inputs=+-
  Bus Selector : BusSelector  OutputSignals=VTQD_PTAvailMotTq_Nm,VTQD_VCUVehSpd_kph
  Bus Selector1 : BusSelector  OutputSignals=VINP_MotorSpd_rpm,VINP_MotorSpdValid_flg,task_time_s,VINP_ECPVCUAcclLim_mps,VINP_CANMsgValidECP2_flg,VINP_ECPVCUAcclLimSw_flg,VINP_FASpeedValid_flg
  Constant1 : Constant  Value=KTQD_VehAccelCalDeltaT_s
  Constant10 : Constant  Value=KTQD_EMSpdAcclLimitEnHi_rpm
  Constant11 : Constant  Value=KTQD_VehAccelCalDeltaT_s
  Constant12 : Constant  Value=KTQD_VehAccelCalFilterTs_s
  Constant13 : Constant  Value=KTQD_VehAccelLimInRagDis_mps2
  Constant14 : Constant  Value=KTQD_VehAccelOvrLimRefreTime_s
  Constant15 : Constant  Value=ENUM_GEARACTUALPOSN_D
  Constant16 : Constant  Value=KTQD_VehAccelOvrLimRefreTime_s
  Constant17 : Constant  Value=KTQD_VehAccelCalEna_kph
  Constant18 : Constant  Value=KTQD_VehAccelLimOvrRagDis_mps2
  Constant19 : Constant  Value=KTQD_VehSpdLimitTorLowerLim_Nm
  Constant2 : Constant  Value=KTQD_VehAcclLimitTG_msp2
  Constant20 : Constant  Value=KTQD_MCUMaxRefTorq_Nm
  Constant21 : Constant  Value=KTQD_VehAcclLimitSW_flg_ovrdflg
  Constant22 : Constant  Value=KTQD_VehAcclLimitSW_flg_ovrdval
  Constant23 : Constant  Value=EPS
  Constant3 : Constant  Value=SINGLEMAXCNT
  Constant4 : Constant  Value=KTQD_VehAcclLimitTG_msp2
  Constant5 : Constant  Value=KTQD_ECPSetValErr1_mps2
  Constant6 : Constant  Value=KTQD_VehAccPhyShrehold_mps2
  Constant7 : Constant  Value=KTQD_ECPSetValNoReq_mps2
  Constant8 : Constant  Value=KTQD_VehAcclLimitExtre_mps2  OutDataTypeStr=single
  Constant9 : Constant  Value=KTQD_EMSpdAcclLimitEnLow_rpm
  Counter1 : hcu_lib/Basic_Blocks/Counter
  Counter2 : hcu_lib/Basic_Blocks/Counter
  Data Type Conversion : DataTypeConversion  OutDataTypeStr=single
  Data Type Conversion1 : DataTypeConversion  OutDataTypeStr=single
  Data Type Conversion2 : DataTypeConversion  OutDataTypeStr=single
  Detect Increase1 : simulink/Logic and Bit Operations/Detect Increase  vinit=boolean(0)  OutDataTypeStr=boolean
  Detect Increase2 : simulink/Logic and Bit Operations/Detect Increase  vinit=boolean(0)  OutDataTypeStr=boolean
  Divide1 : Product  Inputs=*/
  Equal : RelationalOperator  OutDataTypeStr=boolean  RndMeth=Simplest
  Equal1 : RelationalOperator  Operator===  OutDataTypeStr=boolean  RndMeth=Simplest
  Floor : Rounding
  Limit Torque Calaulation : Subsystem  TreatAsAtomicUnit=on
  Limit1 : hcu_lib/Basic_Blocks/Limit
  MTQD_AccelLimitInRange_Z_Gain : Lookup_n-D  BreakpointsForDimension1=ATQD_AccelLimitInRange_Y_Nm  BreakpointsForDimension2=ATQD_AccelLimitInRange_X_rpm  Table=MTQD_AccelLimitInRange_Z_Gain  InternalRulePriority=Speed  RndMeth=Simplest  InputSameDT=on
      settings: InputPortMap=u0,u1
  Max : MinMax  Function=max  Inputs=2
  Min1 : MinMax  Inputs=2
  NOT{,1..4} (5 alike) : Logic  Operator=NOT  AllPortsSameDT=off  OutDataTypeStr=boolean
  OR : Logic  Operator=OR  AllPortsSameDT=off  OutDataTypeStr=boolean
  OR1 : Logic  Operator=OR  AllPortsSameDT=off  OutDataTypeStr=boolean
  OR2 : Logic  Inputs=3  AllPortsSameDT=off  OutDataTypeStr=boolean
  Product2 : Product
  Relational Operator{,4,6..7} (4 alike) : RelationalOperator  OutDataTypeStr=boolean  RndMeth=Simplest
  Relational Operator1 : RelationalOperator  Operator=>  OutDataTypeStr=boolean  RndMeth=Simplest
  Relational Operator13 : RelationalOperator  Operator=<  OutDataTypeStr=boolean  RndMeth=Simplest
  Relational Operator14 : RelationalOperator  Operator=<=  OutDataTypeStr=boolean  RndMeth=Simplest
  Relational Operator5 : RelationalOperator  Operator=>  OutDataTypeStr=boolean  RndMeth=Simplest
  Relational Operator8 : RelationalOperator  Operator=<=  OutDataTypeStr=boolean  RndMeth=Simplest
  SR_Latch : hcu_lib/Basic_Blocks/SR_Latch
  Saturation : Saturate  UpperLimit=KTQD_MCUMaxRefTorq_Nm  LowerLimit=ZERO_FLOAT
      settings: AttributesFormatString=|
      | UpperLimit:%<UpperLimit>
      | LowerLimit:%<LowerLimit>
  Saturation1 : Saturate  UpperLimit=KTQD_EMSpdAcclLimitEnHi_rpm  LowerLimit=ZERO_FLOAT
      settings: AttributesFormatString=|
      | UpperLimit:%<UpperLimit>
      | LowerLimit:%<LowerLimit>
  Switch{1..2,5..9} (7 alike) : Switch  Criteria=u2 ~= 0
      settings: AttributesFormatString=%<Criteria>
  Unit Delay10 : UnitDelay  InitialCondition=boolean(0)  SampleTime=-1  HasFrameUpgradeWarning=on
      settings: AttributesFormatString=%<InitialCondition>
  Unit Delay6 : UnitDelay  InitialCondition=boolean(0)  SampleTime=-1  HasFrameUpgradeWarning=on
      settings: AttributesFormatString=%<InitialCondition>
  Unit Delay8 : UnitDelay  InitialCondition=THOUSAND  SampleTime=-1  HasFrameUpgradeWarning=on
      settings: AttributesFormatString=%<InitialCondition>
  Unit Delay9 : UnitDelay  InitialCondition=single(0)  SampleTime=-1  HasFrameUpgradeWarning=on
      settings: AttributesFormatString=%<InitialCondition>
  Vehicle Acceleration Calculation : Subsystem
  VTQD_VehAcclLimitEnable_flg : Outport
  VTQD_VehAcclLimitTG_mps2 : Outport  Port=2
  VTQD_VehAcclTorLimit_Nm : Outport  Port=3
  VTQD_VehAccel_mps2 : Outport  Port=4
  wires:
  [VTQD_VehAcclLimitEnable_flg] -> VTQD_VehAcclLimitEnable_flg/1
  BSCPIn_outputs/1 -> Bus Selector1/1
  Bus Selector/1 -> [VTQD_PTAvailMotTq_Nm]  "<VTQD_PTAvailMotTq_Nm>"
  BSignalConvert_outputs/1 -> Bus Selector/1
  [VINP_MotorSpdValid_flg] -> OR2/3
  [VINP_MotorSpd_rpm] -> Relational Operator7/1
  Constant10/1 -> Relational Operator8/2
  [VINP_MotorSpd_rpm] -> Relational Operator8/1
  Relational Operator7/1 -> OR2/1
  Constant9/1 -> Relational Operator7/2
  Relational Operator8/1 -> OR2/2
  OR2/1 -> [VTQD_VehAcclEMSpdInRange_flg]  "VTQD_VehAcclEMSpdInRange_flg"
  [VTQD_VehAcclLimitTG_mps2] -> Switch2/1
  [VTQD_VehAcclLimitEnable_flg] -> Switch2/2
  Constant6/1 -> Switch2/3
  Switch2/1 -> [VTQD_VehAcclLimitRef_mps2]  "VTQD_VehAcclLimitRef_mps2"
  Relational Operator1/1 -> [VTQD_VehAcceleOvrRef_flg]  "VTQD_VehAcceleOvrRef_flg"
  [VTQD_VehAccel_mps2] -> Relational Operator1/1
  Constant18/1 -> Add1/2
  [VTQD_VehAccel_mps2] -> Relational Operator4/1
  [VTQD_VehAccel_mps2] -> Relational Operator5/1
  Add6/1 -> Relational Operator4/2
  Relational Operator4/1 -> [VTQD_VehAcceleInLimit_flg]  "VTQD_VehAcceleInLimit_flg"
  Add1/1 -> Relational Operator5/2
  [VTQD_VehAcclLimitRef_mps2] -> Add1/1
  [VTQD_VehAcclLimitRef_mps2] -> Add6/1
  Constant13/1 -> Add6/2
  Relational Operator5/1 -> [VTQD_VehAcceleOvrLimit_flg]  "VTQD_VehAcceleOvrLimit_flg"
  [VTQD_VehAcclLimitRef_mps2] -> Relational Operator1/2
  Counter2/1 -> Equal/1
  Relational Operator/1 -> NOT/1, Counter2/1
  OR/1 -> Unit Delay10/1
  Divide1/1 -> Floor/1
  Unit Delay10/1 -> Counter2/2
  Equal/1 -> [VTQD_VehAccelCalTrig_flg]  "VTQD_VehAccelCalTrig_flg"
  [VTQD_VCUVehSpd_kph] -> Relational Operator/1
  NOT/1 -> OR/1
  Constant17/1 -> Relational Operator/2
  [VTQD_VehAccelCalTrig_flg] -> OR/2
  [VTQD_VehAcceleOvrLimit_flg] -> NOT2/1, Counter1/1
  NOT2/1 -> OR1/1
  OR1/1 -> Counter1/2
  Relational Operator6/1 -> [VTQD_VehAcceleContiOvrLimit_flg], Unit Delay6/1  "VTQD_VehAcceleContiOvrLimit_flg"
  Unit Delay6/1 -> OR1/2
  Counter1/1 -> Product2/1
  Constant14/1 -> Relational Operator6/2
  Product2/1 -> Relational Operator6/1
  Constant3/1 -> Counter1/3
  [task_time_s] -> Product2/2
  Switch1/1 -> AND3/7
  NOT1/1 -> AND3/3
  Constant15/1 -> Equal1/2
  [VTQD_VehAcclEMSpdInRange_flg] -> AND3/4
  Constant21/1 -> Switch1/2
  [VTQD_GearActualPosn_enum] -> Equal1/1
  [VINP_ECPVCUAcclLim_mps] -> Relational Operator13/1
  Relational Operator13/1 -> AND3/6
  Constant22/1 -> Switch1/1
  Equal1/1 -> AND3/1
  [VINP_ECPVCUAcclLimSw_flg] -> NOT1/1
  [VINP_CANMsgValidECP2_flg] -> AND3/2
  [VINP_FASpeedValid_flg] -> AND3/5
  Constant5/1 -> Relational Operator13/2
  AND3/1 -> [VTQD_VehAcclLimitEnable_flg]  "VTQD_VehAcclLimitEnable_flg"
  [VTQD_VCUVehSpd_kph] -> Vehicle Acceleration Calculation/1(VTQD_VCUVehSpd_kph)
  Constant12/1 -> Vehicle Acceleration Calculation/4(KTQD_VehAccelCalFilterTs_s)
  [task_time_s] -> Vehicle Acceleration Calculation/2(VTQD_tasktime_s)
  Vehicle Acceleration Calculation/1(VTQD_VehAccel_mps2) -> Data Type Conversion2/1
  [VTQD_VehAccelCalTrig_flg] -> Vehicle Acceleration Calculation/Trigger
  Constant7/1 -> Relational Operator14/2
  Min1/1 -> Switch9/1
  [VINP_ECPVCUAcclLim_mps] -> Relational Operator14/1
  [VTQD_VehAcclLimitEnable_flg] -> Switch9/2
  Switch5/1 -> Min1/2
  [VINP_ECPVCUAcclLim_mps] -> Switch5/3
  Relational Operator14/1 -> Switch5/2
  Switch9/1 -> [VTQD_VehAcclLimitTG_mps2]  "VTQD_VehAcclLimitTG_mps2"
  Constant8/1 -> Switch9/3
  Limit Torque Calaulation/1(Result) -> Data Type Conversion/1
  Data Type Conversion/1 -> Switch8/1
  [VTQD_VehAcceleOvrRef_flg] -> NOT3/1
  [VTQD_VehAcceleContiOvrLimit_flg] -> Limit Torque Calaulation/Trigger
  Detect Increase2/1 -> Switch6/2
  [VTQD_VehAcceleInLimit_flg] -> Detect Increase1/1
  NOT3/1 -> SR_Latch/2
  NOT4/1 -> Switch7/2
  [VINP_MotorSpd_rpm] -> Saturation1/1
  [VTQD_VehAccel_mps2] -> Limit Torque Calaulation/2(VehAccel)
  Saturation/1 -> MTQD_AccelLimitInRange_Z_Gain/1
  SR_Latch/1 -> NOT4/1
  Detect Increase1/1 -> SR_Latch/1
  Saturation1/1 -> MTQD_AccelLimitInRange_Z_Gain/2
  [VTQD_VehAcceleInLimit_flg] -> Detect Increase2/1
  Limit1/1 -> [VTQD_VehAcclTorLimit_Nm]  "VTQD_VehAcclTorLimit_Nm"
  MTQD_AccelLimitInRange_Z_Gain/1 -> Switch6/1
  Constant16/1 -> Limit Torque Calaulation/3(PIControl_Task_time)
  Unit Delay8/1 -> Switch7/3
  [VTQD_PedalMapTq_Nm] -> Saturation/1
  [VTQD_VehAcclTorLimit_Nm] -> Unit Delay8/1
  [VTQD_VehAcclTorLimit_Nm] -> Unit Delay9/1
  Switch6/1 -> Switch8/3
  Constant19/1 -> Limit1/3
  Switch8/1 -> Limit1/1
  Switch7/1 -> Switch6/3
  Unit Delay9/1 -> Limit Torque Calaulation/4(VTQD_VehAccelTorLimitLast_Nm)
  Constant20/1 -> Limit1/2
  [VTQD_VehAcceleContiOvrLimit_flg] -> Switch8/2
  [VTQD_PTAvailMotTq_Nm] -> Switch7/1
  [VTQD_VehAcclLimitRef_mps2] -> Limit Torque Calaulation/1(Refference)
  Constant1/1 -> Divide1/1
  Constant2/1 -> Switch5/1
  Constant4/1 -> Min1/1
  VTQD_GearActualPosn_enum/1 -> [VTQD_GearActualPosn_enum]
  [VINP_ECPVCUAcclLimSw_flg] -> Switch1/3
  Constant11/1 -> Vehicle Acceleration Calculation/3(KTQD_VehAccelCalDeltaT_s)
  VTQD_PedalMapTq_Nm/1 -> [VTQD_PedalMapTq_Nm]
  [VTQD_VehAcclLimitTG_mps2] -> VTQD_VehAcclLimitTG_mps2/1
  [VTQD_VehAcclTorLimit_Nm] -> VTQD_VehAcclTorLimit_Nm/1
  [VTQD_VehAccel_mps2] -> VTQD_VehAccel_mps2/1
  Max/1 -> Divide1/2
  [task_time_s] -> Max/1
  Constant23/1 -> Max/2
  Floor/1 -> Data Type Conversion1/1
  Data Type Conversion2/1 -> [VTQD_VehAccel_mps2]  "VTQD_VehAccel_mps2"
  Data Type Conversion1/1 -> Equal/2, Counter2/3  "VTQD_VehAccelCalDeltaT_cnt"
  Bus Selector1/1 -> [VINP_MotorSpd_rpm]  "<VINP_MotorSpd_rpm>"
  Bus Selector1/2 -> [VINP_MotorSpdValid_flg]  "<VINP_MotorSpdValid_flg>"
  Bus Selector1/3 -> [task_time_s]  "<task_time_s>"
  Bus Selector1/4 -> [VINP_ECPVCUAcclLim_mps]  "<VINP_ECPVCUAcclLim_mps>"
  Bus Selector1/5 -> [VINP_CANMsgValidECP2_flg]  "<VINP_CANMsgValidECP2_flg>"
  Bus Selector1/6 -> [VINP_ECPVCUAcclLimSw_flg]  "<VINP_ECPVCUAcclLimSw_flg>"
  Bus Selector1/7 -> [VINP_FASpeedValid_flg]  "<VINP_FASpeedValid_flg>"
  Bus Selector/2 -> [VTQD_VCUVehSpd_kph]  "<VTQD_VCUVehSpd_kph>"

== system tqd/TQD/Input_Convert/Function/BOS ==
  BSCPIn_outputs : Inport
  BSignalConvert_outputs : Inport  Port=2
  VTQD_GearActualPosn_enum : Inport  Port=3
  VTQD_PedalMapTq_Nm : Inport  Port=4
  Bus Selector : BusSelector  OutputSignals=VTQD_TqTargetShaftSpd_rpm
  Bus Selector1 : BusSelector  OutputSignals=VINP_BrakePedalPos_pct
  Constant1 : Constant  Value=ENUM_GEARACTUALPOSN_R
  Constant2 : Constant  Value=ZERO_FLOAT
  Constant3 : Constant  Value=HUNDRED
  Equal : RelationalOperator  Operator===  OutDataTypeStr=boolean  RndMeth=Simplest
  MTQD_BOSMapD_Z_pct : Lookup_n-D  BreakpointsForDimension1=ATQD_BOSMapD_Y_pct  BreakpointsForDimension2=ATQD_BOSMapD_X_rpm  Table=MTQD_BOSMapD_Z_pct  InternalRulePriority=Speed  RndMeth=Simplest  InputSameDT=on
      settings: InputPortMap=u0,u1
  MTQD_BOSMapR_Z_pct : Lookup_n-D  BreakpointsForDimension1=ATQD_BOSMapR_Y_pct  BreakpointsForDimension2=ATQD_BOSMapR_X_rpm  Table=MTQD_BOSMapR_Z_pct  InternalRulePriority=Speed  RndMeth=Simplest  InputSameDT=on
      settings: InputPortMap=u0,u1
  Relational Operator : RelationalOperator  OutDataTypeStr=boolean  RndMeth=Simplest
  Switch : Switch  Criteria=u2 ~= 0
      settings: AttributesFormatString=%<Criteria>
  Switch1 : Switch  Criteria=u2 ~= 0
      settings: AttributesFormatString=%<Criteria>
  VTQD_BOSTqDecRate_pct : Outport
  wires:
  [VTQD_BOSTqDecRate_pct] -> VTQD_BOSTqDecRate_pct/1
  Bus Selector1/1 -> [VINP_BrakePedalPos_pct]  "<VINP_BrakePedalPos_pct>"
  BSCPIn_outputs/1 -> Bus Selector1/1
  Bus Selector/1 -> [VTQD_TqTargetShaftSpd_rpm]  "<VTQD_TqTargetShaftSpd_rpm>"
  BSignalConvert_outputs/1 -> Bus Selector/1
  [VINP_BrakePedalPos_pct] -> MTQD_BOSMapD_Z_pct/1
  [VTQD_TqTargetShaftSpd_rpm] -> MTQD_BOSMapD_Z_pct/2
  [VTQD_TqTargetShaftSpd_rpm] -> MTQD_BOSMapR_Z_pct/2
  [VINP_BrakePedalPos_pct] -> MTQD_BOSMapR_Z_pct/1
  [VTQD_GearActualPosn_enum] -> Equal/1
  Constant1/1 -> Equal/2
  Equal/1 -> Switch/2
  MTQD_BOSMapR_Z_pct/1 -> Switch/1
  MTQD_BOSMapD_Z_pct/1 -> Switch/3
  VTQD_GearActualPosn_enum/1 -> [VTQD_GearActualPosn_enum]
  Switch/1 -> Switch1/1
  VTQD_PedalMapTq_Nm/1 -> [VTQD_PedalMapTq_Nm]
  Relational Operator/1 -> Switch1/2
  [VTQD_PedalMapTq_Nm] -> Relational Operator/1
  Constant2/1 -> Relational Operator/2
  Constant3/1 -> Switch1/3
  Switch1/1 -> [VTQD_BOSTqDecRate_pct]  "VTQD_BOSTqDecRate_pct"
